simulink model "Simple_LQR"  (R2019a)
settings: Solver=VariableStepAuto  StartTime=0.0  StopTime=10.0  RelTol=1e-3
settings Model: Creator=martin  LastModifiedBy=martin

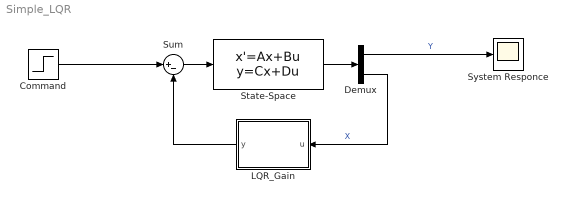
== system Simple_LQR ==
  Command : Step  SampleTime=0
  Demux : Demux  Outputs=2
  LQR_Gain : MATLAB Function  TreatAsAtomicUnit=on
  State-Space : StateSpace  InitialCondition=0
  Sum : Sum  Inputs=|+-
  System Responce : Scope
  wires:
  State-Space/1 -> Demux/1
  Demux/1 -> System Responce/1  "Y"
  Demux/2 -> LQR_Gain/1(u)  "X"
  LQR_Gain/1(y) -> Sum/2
  Sum/1 -> State-Space/1
  Command/1 -> Sum/1

== matlab function Simple_LQR/LQR_Gain ==
  data: u input; y output
function y = fcn(u)

y = u;
